simulink model "TorqueVectoringAllocator"  (R2026b)
settings: Solver=FixedStepDiscrete  StopTime=1.0  FixedStep=TorqueVectoringControlSampleTime
settings Model: DataDictionary=VehicleData.sldd  Creator=Xu Dingyi  LastModifiedBy=29358
settings DebuggingCC: AlgebraicLoopMsg=error

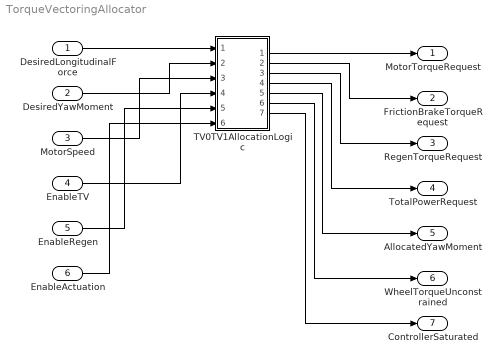
== system TorqueVectoringAllocator ==
  DesiredLongitudinalForce : Inport  OutDataTypeStr=double  Unit=N
  DesiredYawMoment : Inport  Port=2  OutDataTypeStr=double  Unit=N*m
  MotorSpeed : Inport  Port=3  OutDataTypeStr=double  Unit=rad/s  PortDimensions=4
  EnableTV : Inport  Port=4  OutDataTypeStr=boolean
  EnableRegen : Inport  Port=5  OutDataTypeStr=boolean
  EnableActuation : Inport  Port=6  OutDataTypeStr=boolean
  TV0TV1AllocationLogic : Stateflow chart  TreatAsAtomicUnit=on
  MotorTorqueRequest : Outport  OutDataTypeStr=double  Unit=N*m  PortDimensions=4
  FrictionBrakeTorqueRequest : Outport  Port=2  OutDataTypeStr=double  Unit=N*m  PortDimensions=4
  RegenTorqueRequest : Outport  Port=3  OutDataTypeStr=double  Unit=N*m  PortDimensions=4
  TotalPowerRequest : Outport  Port=4  OutDataTypeStr=double  Unit=W
  AllocatedYawMoment : Outport  Port=5  OutDataTypeStr=double  Unit=N*m
  WheelTorqueUnconstrained : Outport  Port=6  OutDataTypeStr=double  Unit=N*m  PortDimensions=4
  ControllerSaturated : Outport  Port=7  OutDataTypeStr=boolean
  wires:
  MotorSpeed/1 -> TV0TV1AllocationLogic/3(MotorSpeed)
  EnableActuation/1 -> TV0TV1AllocationLogic/6(EnableActuation)
  DesiredYawMoment/1 -> TV0TV1AllocationLogic/2(DesiredYawMoment)
  EnableRegen/1 -> TV0TV1AllocationLogic/5(EnableRegen)
  EnableTV/1 -> TV0TV1AllocationLogic/4(EnableTV)
  DesiredLongitudinalForce/1 -> TV0TV1AllocationLogic/1(DesiredLongitudinalForce)
  TV0TV1AllocationLogic/1(MotorTorqueRequest) -> MotorTorqueRequest/1
  TV0TV1AllocationLogic/2(FrictionBrakeTorqueRequest) -> FrictionBrakeTorqueRequest/1
  TV0TV1AllocationLogic/3(RegenTorqueRequest) -> RegenTorqueRequest/1
  TV0TV1AllocationLogic/4(TotalPowerRequest) -> TotalPowerRequest/1
  TV0TV1AllocationLogic/5(AllocatedYawMoment) -> AllocatedYawMoment/1
  TV0TV1AllocationLogic/6(WheelTorqueUnconstrained) -> WheelTorqueUnconstrained/1
  TV0TV1AllocationLogic/7(ControllerSaturated) -> ControllerSaturated/1

== stateflow chart TorqueVectoringAllocator/TV0TV1AllocationLogic ==
  state Allocate
    du: [MotorTorqueRequest, FrictionBrakeTorqueRequest, RegenTorqueRequest, TotalPowerRequest, AllocatedYawMoment, WheelTorqueUnconstrained, ControllerSaturated] = torqueVectoringAllocateWheelTorque(DesiredLongitudinalForce, DesiredYawMoment, MotorSpeed, EnableTV, EnableRegen, EnableActuation, TorqueVectoringTireEffectiveRadius, TorqueVectoringGearRatio, TorqueVectoringGearEfficiency, TorqueVectoringMotorTorqueLimit, TorqueVectoringMotorSpeedLimit, TorqueVectoringInverterEfficiency, TorqueVectoringDrivePowerLimit, TorqueVectoringRegenPowerLimit, TorqueVectoringTrackFront, TorqueVectoringTrackRear, TorqueVectoringBrakeMaxTorque, TorqueVectoringPowerEpsilon);
  (default) -> Allocate
  data: DesiredLongitudinalForce input double; DesiredYawMoment input double; MotorSpeed input double; EnableTV input boolean; EnableRegen input boolean; EnableActuation input boolean; MotorTorqueRequest output double; FrictionBrakeTorqueRequest output double; RegenTorqueRequest output double; TotalPowerRequest output double; AllocatedYawMoment output double; WheelTorqueUnconstrained output double; ControllerSaturated output boolean; TorqueVectoringTireEffectiveRadius parameter double; TorqueVectoringGearRatio parameter double; TorqueVectoringGearEfficiency parameter double; TorqueVectoringMotorTorqueLimit parameter double; TorqueVectoringMotorSpeedLimit parameter double; TorqueVectoringInverterEfficiency parameter double; TorqueVectoringDrivePowerLimit parameter double; TorqueVectoringRegenPowerLimit parameter double; TorqueVectoringTrackFront parameter double; TorqueVectoringTrackRear parameter double; TorqueVectoringBrakeMaxTorque parameter double; TorqueVectoringPowerEpsilon parameter double
